simulink model "acc_settings"  (R2021a)
settings: Solver=FixedStepAuto  StartTime=0.0  StopTime=inf  FixedStep=2.0  RelTol=1e-3
libraries: robotlib x9
settings Model: Creator=ivory  LastModifiedBy=refulgent
settings SolverCC: AlgebraicLoopSolver=TrustRegion
settings OptimizationCC: EnhancedBackFolding=on  PassReuseOutputArgsAs=Individual arguments  ZeroExternalMemoryAtStartup=off  ZeroInternalMemoryAtStartup=off  MaxStackSize=64  OptimizeBlockOrder=speed  DifferentSizesBufferReuse=on  OptimizationCustomize=off  EfficientTunableParamExpr=on
settings DebuggingCC: ParameterTunabilityLossMsg=error  SFMachineParentedDataDiag=warning
settings HardwareCC: ProdBitPerPointer=32  ProdBitPerSizeT=32  ProdBitPerPtrDiffT=32  ProdLargestAtomicFloat=None  ProdIntDivRoundTo=Undefined  ProdEndianess=Unspecified  ProdWordSize=32  ProdHWDeviceType=Generic->Unspecified (assume 32-bit Generic)
settings SFSimCC: MATLABDynamicMemAlloc=off  SimTargetLang=C++
settings RTWCC: SystemTargetFile=ert.tlc  HardwareBoard=Robot Operating System (ROS)  TLCOptions="-aInlineSetEventsForThisBaseRateFcn=TLC_FALSE -aSuppressMultiTaskScheduler=TLC_FALSE  -aRateBasedStepFcn=0"  TemplateMakefile=ert_default_tmf  GenerateReport=on  Toolchain=Catkin  IncludeHyperlinkInReport=on  LaunchReport=on  TargetLang=C++  GenerateTraceInfo=on  GenerateTraceReport=on  GenerateTraceReportSl=on  GenerateTraceReportSf=on  GenerateTraceReportEml=on
settings CodeAppCC: ForceParamTrailComments=on  IgnoreCustomStorageClasses=off  OperatorAnnotations=on  SimulinkDataObjDesc=on  SFDataObjDesc=on  InsertBlockDesc=on
settings ERTTargetCC: SupportContinuousTime=on  SupportVariableSizeSignals=on

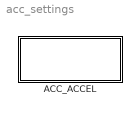
== system acc_settings ==
  ACC_ACCEL : Subsystem

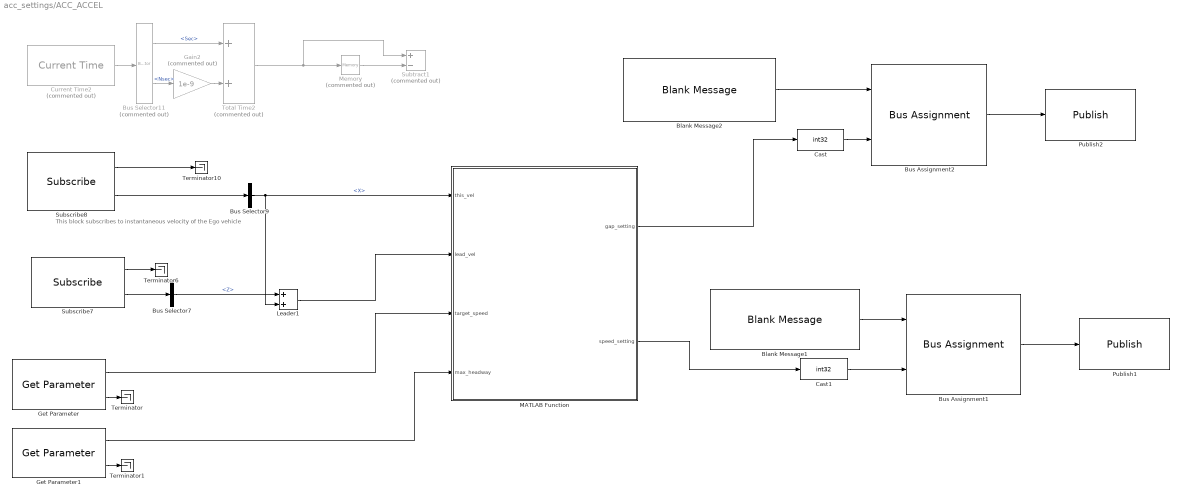
== system acc_settings/ACC_ACCEL ==
  note: This block subscribes to
      | instantaneous velocity of the Ego vehicle
  Blank Message1 : robotlib/Blank Message  messageClass=Message  entityType=std_msgs/Int32  messageType=std_msgs/Int32  SampleTime=inf  legacyBusStruct=off
  Blank Message2 : robotlib/Blank Message  messageClass=Message  entityType=std_msgs/Int32  messageType=std_msgs/Int32  SampleTime=inf  legacyBusStruct=off
  Bus Assignment1 : BusAssignment  AssignedSignals=Data
  Bus Assignment2 : BusAssignment  AssignedSignals=Data
  Bus Selector11 : BusSelector  Commented=on  OutputSignals=Sec,Nsec
  Bus Selector7 : BusSelector  OutputSignals=Linear.Z
  Bus Selector9 : BusSelector  OutputSignals=Linear.X
  Cast : DataTypeConversion  OutDataTypeStr=int32
  Cast1 : DataTypeConversion  OutDataTypeStr=int32
  Current Time2 : robotlib/Current Time  Commented=on  OutputFormat=bus  SampleTime=-1  ModelName=microaccel
      settings: SourceProductBaseCode=RR
  Gain2 : Gain  Commented=on  Gain=1e-9
  Get Parameter : robotlib/Get Parameter  ParameterSource=Specify your own  ParameterName=target_speed  ParameterType=double  ParameterMaxArrayLength=16  ParameterInitialValue=25.0  SampleTime=-1  ShowErrorCodeOutput=on  ModelName=acc_accel  BlockId=ParamGet_acc_accel_655
      settings: SourceProductBaseCode=RR
  Get Parameter1 : robotlib/Get Parameter  ParameterSource=Specify your own  ParameterName=max_headway  ParameterType=double  ParameterMaxArrayLength=16  ParameterInitialValue=50.0  SampleTime=-1  ShowErrorCodeOutput=on  ModelName=acc_accel  BlockId=ParamGet_acc_accel_657
      settings: SourceProductBaseCode=RR
  Leader1 : Sum
  MATLAB Function : MATLAB Function  TreatAsAtomicUnit=on
  Memory : Memory  Commented=on
  Publish1 : robotlib/Publish  topicSource=Specify your own  topic=speed_setting  messageType=std_msgs/Int32  legacyBusStruct=off  messageQueueLength=1
  Publish2 : robotlib/Publish  topicSource=Specify your own  topic=gap_setting  messageType=std_msgs/Int32  legacyBusStruct=off  messageQueueLength=1
  Subscribe7 : robotlib/Subscribe  topicSource=Specify your own  topic=rel_vel  messageType=geometry_msgs/Twist  SampleTime=-1  legacyBusStruct=off  messageQueueLength=1
  Subscribe8 : robotlib/Subscribe  topicSource=Specify your own  topic=vel  messageType=geometry_msgs/Twist  SampleTime=-1  legacyBusStruct=off  messageQueueLength=1
  Subtract1 : Sum  Commented=on  Inputs=+-
  Terminator{,1,6,10} (4 alike) : Terminator
  Total Time2 : Sum  Commented=on
  wires:
  Bus Selector11/1 -> Total Time2/1  "<Sec>"
  Gain2/1 -> Total Time2/2
  Bus Selector11/2 -> Gain2/1  "<Nsec>"
  Total Time2/1 -> Subtract1/1, Memory/1
  Current Time2/1 -> Bus Selector11/1
  Memory/1 -> Subtract1/2
  Subscribe8/2 -> Bus Selector9/1
  Subscribe8/1 -> Terminator10/1
  Bus Selector9/1 -> MATLAB Function/1(this_vel), Leader1/2  "<X>"
  Bus Selector7/1 -> Leader1/1  "<Z>"
  Subscribe7/1 -> Terminator6/1
  Subscribe7/2 -> Bus Selector7/1
  Leader1/1 -> MATLAB Function/2(lead_vel)
  Get Parameter/1 -> MATLAB Function/3(target_speed)
  Get Parameter/2 -> Terminator/1
  Get Parameter1/2 -> Terminator1/1
  Get Parameter1/1 -> MATLAB Function/4(max_headway)
  Bus Assignment2/1 -> Publish2/1
  Blank Message2/1 -> Bus Assignment2/1
  MATLAB Function/1(gap_setting) -> Cast/1
  MATLAB Function/2(speed_setting) -> Cast1/1
  Blank Message1/1 -> Bus Assignment1/1
  Bus Assignment1/1 -> Publish1/1
  Cast/1 -> Bus Assignment2/2
  Cast1/1 -> Bus Assignment1/2

== matlab function acc_settings/ACC_ACCEL/MATLAB Function ==
  settings: updateMethod=DISCRETE
  data: this_vel input; lead_vel input; gap_setting output; target_speed input; max_headway input; speed_setting output
function [gap_setting, speed_setting] =  get_acc_accel(this_vel, lead_vel, target_speed, max_headway)
        %%"""See parent class."""
        % TODO (Eugene, Nathan, Adit, Fahd, Kathy): replace with trained controller
        MPH_TO_MS = 0.44704;
        if target_speed == -1
            if lead_vel < 20 * MPH_TO_MS
                speed_setting = lead_vel;
                if abs(this_vel - lead_vel) < 2.0
                    gap_setting = 2;
                elseif this_vel > lead_vel
                    gap_setting = 1;
                else
                    gap_setting = 3;
                end
            else
                if this_vel > lead_vel + 2
                    gap_setting = 1;
                    speed_setting = lead_vel;
                else
                    gap_setting = 3;
                    speed_setting = (this_vel + lead_vel) / 2.0;
                end
            end
        else
            if target_speed < lead_vel
                speed_setting = target_speed*0.6 + lead_vel*0.4;
            else
                speed_setting = target_speed;
            end
            if max_headway
                gap_setting = 1;
            else
                gap_setting = 3;
            end
        end
        speed_setting = max(speed_setting, MPH_TO_MS * 20);
%         speed_setting =int(round(speed_setting));
%         gap_setting = int(gap_setting);
%         accel = get_accel(this_vel, lead_vel, headway, speed_setting, time_gap_setting=gap_setting);
%         self.accel_without_noise = accel;
end
